simulink model "formation_control_alternative_tanks"  (R2021a)
settings: Solver=VariableStepAuto  StartTime=0.0  StopTime=T  RelTol=1e-3
undefined symbols (not defined in the file or in its folder): params
settings Model: Creator=gaeta  LastModifiedBy=giuse
settings SolverCC: AlgebraicLoopSolver=TrustRegion
settings DataIOCC: InitialState=initialCondition  LoadInitialState=on
settings DebuggingCC: SFMachineParentedDataDiag=warning

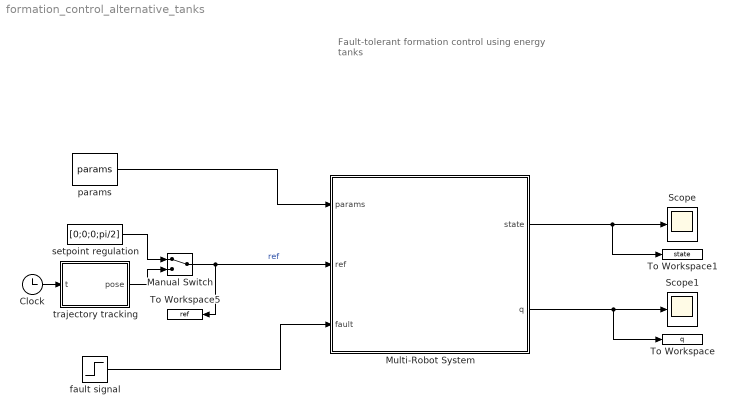
== system formation_control_alternative_tanks ==
  note: Fault-tolerant formation control
      | using energy tanks
  Clock : Clock
  Manual Switch : ManualSwitch
  Multi-Robot System : Subsystem
  Scope : Scope
  Scope1 : Scope
  To Workspace : ToWorkspace  VariableName=q  SaveFormat=Timeseries  SampleTime=-1
  To Workspace1 : ToWorkspace  VariableName=state  SaveFormat=Timeseries  SampleTime=-1
  To Workspace5 : ToWorkspace  VariableName=ref  SaveFormat=Timeseries  SampleTime=-1
  fault signal : Step  Time=25  SampleTime=0
  params : Constant  Value=params  OutDataTypeStr=Bus: params_bus
  setpoint regulation : Constant  Value=[0;0;0;pi/2]
  trajectory tracking : MATLAB Function  TreatAsAtomicUnit=on
  wires:
  trajectory tracking/1(pose) -> Manual Switch/2
  setpoint regulation/1 -> Manual Switch/1
  Clock/1 -> trajectory tracking/1(t)
  Manual Switch/1 -> To Workspace5/1, Multi-Robot System/2(ref)  "ref"
  Multi-Robot System/2(q) -> Scope1/1, To Workspace/1
  Multi-Robot System/1(state) -> Scope/1, To Workspace1/1
  params/1 -> Multi-Robot System/1(params)
  fault signal/1 -> Multi-Robot System/3(fault)

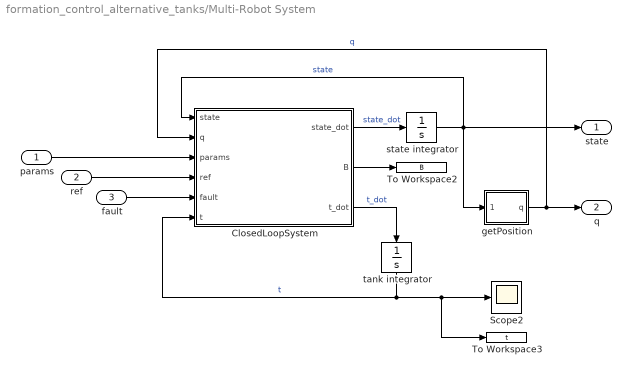
== system formation_control_alternative_tanks/Multi-Robot System ==
  params : Inport
  ref : Inport  Port=2
  fault : Inport  Port=3
  ClosedLoopSystem : MATLAB Function  TreatAsAtomicUnit=on
  Scope2 : Scope
  To Workspace2 : ToWorkspace  VariableName=B  SaveFormat=Timeseries  SampleTime=-1
  To Workspace3 : ToWorkspace  VariableName=t  SaveFormat=Timeseries  SampleTime=-1
  getPosition : Subsystem
  state integrator : Integrator
  tank integrator : Integrator
  state : Outport
  q : Outport  Port=2
  wires:
  ClosedLoopSystem/3(t_dot) -> tank integrator/1  "t_dot"
  getPosition/1(q) -> q/1, ClosedLoopSystem/2(q)  "q"
  ref/1 -> ClosedLoopSystem/4(ref)
  state integrator/1 -> state/1, ClosedLoopSystem/1(state), getPosition/1(state)  "state"
  ClosedLoopSystem/2(B) -> To Workspace2/1
  ClosedLoopSystem/1(state_dot) -> state integrator/1  "state_dot"
  tank integrator/1 -> To Workspace3/1, Scope2/1, ClosedLoopSystem/6(t)  "t"
  fault/1 -> ClosedLoopSystem/5(fault)
  params/1 -> ClosedLoopSystem/3(params)

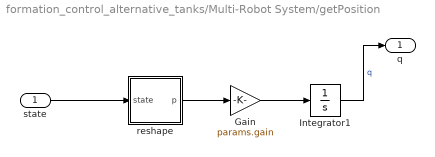
== system formation_control_alternative_tanks/Multi-Robot System/getPosition ==
  state : Inport
  Gain : Gain  Gain=params.gain
  Integrator1 : Integrator
  reshape : MATLAB Function  TreatAsAtomicUnit=on
  q : Outport
  wires:
  state/1 -> reshape/1(state)
  reshape/1(p) -> Gain/1
  Gain/1 -> Integrator1/1
  Integrator1/1 -> q/1  "q"

== matlab function formation_control_alternative_tanks/trajectory tracking ==
  data: pose output size=4; t input size=1
%% generate reference trajectory
function pose = trajectory(t)
t1 = 5;
t_end = 55;

w = 0.25;
phi = -w*t1;
A = 80;
z_vel = 1;

if(t<t1)
    y = [0;0;0];
    theta = pi/2;
elseif(t>t_end)
    y = [A*sin(w*t_end+phi); -A*cos(w*t_end+phi); z_vel*t_end] - [A*sin(w*t1+phi); -A*cos(w*t1+phi); z_vel*t1];
    theta = atan2(A*sin(w*t_end+phi), A*cos(w*t_end+phi));
else
    y = [A*sin(w*t+phi); -A*cos(w*t+phi); z_vel*t] - [A*sin(w*t1+phi); -A*cos(w*t1+phi); z_vel*t1];
    theta = atan2(A*sin(w*t+phi), A*cos(w*t+phi));
end

pose = [y; theta];
end

== matlab function formation_control_alternative_tanks/Multi-Robot System/ClosedLoopSystem ==
  data: state input size=3*(params.N+params.E); q input size=3*params.N; state_dot output size=3*(params.N+params.E); params input; ref input size=4; fault input; t input size=params.N; B output; t_dot output size=params.N
function [state_dot,B,t_dot] = closedLoopSystem(state, q, params, ref, fault, t)
n = 3;	% task space
N = 5;  % number of robots
faulted_robot = params.faulted_robot;
alpha = zeros(N,1);

%% initialize some matrices
p = state(1:n*N);           % robots momenta
m = params.m;               % robots masses
M = zeros(n*N, n*N);      	% inertia matrix
d = params.d;               % frict. coeff
D = zeros(n*N, n*N);        % system dissipation matrix
for i = 1:N
    M(n*i-n+1:n*i, n*i-n+1:n*i) = eye(n).*m(i);
    D(n*i-n+1:n*i, n*i-n+1:n*i) = eye(n).*d(i);
end

%% Check whether a fault is occurred
if(sum(fault)~=0 && ~params.fault_occurred)
    params.fault_occurred = 1;  % flag on
    params.B = faultHandler(params.B, params.Bfull, faulted_robot);
end

%% Still initialize matrices
E = params.E;               % number of edges
B = params.B;
Bcl = kron(params.B,eye(n));% closed-loop incidence matrix
dc = params.dc;             % robots dissipations
Dc = zeros(n*E, n*E);       % controller dissipation matrix
kc = params.kc;             % constant springs
Kc = zeros(n*E, n*E);       % constant spring matrix
R = zeros(n*E, n*E);        % n*E matrix containing E rotation matrices

for j = 1:E
    Dc(n*j-n+1:n*j, n*j-n+1:n*j) = eye(n).*dc(j);
    Kc(n*j-n+1:n*j, n*j-n+1:n*j) = eye(n).*kc(j);
    R(n*j-n+1:n*j, n*j-n+1:n*j) = rotz(ref(4)-pi/2);
end

z = state(n*N+1:n*(N+E));	% edges lengths
z_des = R*params.z_des;     % desired edges lengths

% NOTE: constant matrices M, D, Dc, Kc should be moved in the Init file

%% Trajectory Tracking / Setpoint Regulation
tracking = true;    % #CHANGE THIS: ENABLE/DISABLE TRAJECTORY TRACKING
u = zeros(n*N,1);
if(tracking) 
    % control for leader trajectory tracking
    Kp = 20;
    u(1:n) = Kp*(ref(1:n)-q(1:n));
    
    % control for faulted robot
    K_pd = 0.4;
    P_action = K_pd*(1-q(n*faulted_robot));
	D_action = K_pd*p(n*faulted_robot)/m(faulted_robot);
    u(n*faulted_robot) = params.fault_occurred*(P_action-D_action);
end

%% Multi-robot System Dynamics
Fe = -Bcl * Kc*(z-z_des);           % external forces (control action)
Fa = -(Bcl*Dc*Bcl.')*(M^(-1)*p);	% interaction (coupling) forces
p_dot = Fa + Fe - D*(M^(-1)*p) + u;

% dissipated energy stored in tanks
dissipated_storage = zeros(N,1);
for i = 1:N
    if t(i) >= params.tank_max
        alpha(i) = 0;
    else
        alpha(i) = 1;
    end
    p_i = p(n*i-n+1:i*n);
    M_i = M(n*i-n+1:i*n, n*i-n+1:i*n);
    D_i = D(n*i-n+1:i*n, n*i-n+1:i*n);
    dissipated_storage(i) = alpha(i)*( 1/(t(i)) * ( p_i.' * inv(M_i.') * D_i * inv(M_i) * p_i ) );   
end

% interaction forcess
F = zeros(n,E);
for e = 1:E
    if(isConnected(e,B))
        F(:,e) = kc(e)*( z(n*e-n+1:e*n) - z_des(n*e-n+1:e*n) ); % store force exchanged in edge e-th
    else
        F(:,e) = zeros(n,1);
    end
end

%% Energy transfer protocol
gamma = params.gamma;
t_dot = zeros(N,1);
for i = 1:N
    energy_exchange_tank = 0;
    for e = 1:E
        energy_exchange_tank = energy_exchange_tank + B(i,e)*gamma(e)*t(i)*(F(:,e).'*F(:,e));
    end
    t_dot(i) = dissipated_storage(i) + alpha(i)*energy_exchange_tank;
end

z_dot_a = Bcl.'*(M^(-1)*p);
z_dot_b = zeros(E*n,1);
for e = 1:E
    energy_exchange_spring = zeros(n,1);
    for i = 1:N
        energy_exchange_spring = energy_exchange_spring - B(i,e)*gamma(i)*t(i)^2*F(:,e);
    end
    z_dot_b(e*n-n+1:e*n) = energy_exchange_spring;
end

z_dot = z_dot_a + z_dot_b;

state_dot = [p_dot; z_dot];
end


%% Energy function ----------------------------------------------
function v = V(error)
if (error<=0)
    v = error^2;
elseif(error>=0 && error<5*pi)
    v = 50*cos(0.2*error-pi)+50;
else
    v = 100;
end
end

%% Derivative of the energy function
function vdot = Vdot(error)
if (error<=0)
    vdot = 2*error;
elseif(error>0 && error<5*pi)
    vdot = 10*sin(0.2*error);
else
    vdot = 0;
end
end

%% Split & Join operations
function B = faultHandler(B, Bfull, faulted_robot)
% split procedure
if(faulted_robot==1)
    disp("leader cannot be faulted by hypothesis");
else
    faulted_edges = getEdges(faulted_robot, B);
    for e = 1:size(B,2)
        if(ismember(e,faulted_edges))
           B(:,e) = zeros(size(B,1),1); 
        end
    end
end

% join procedure
if(faulted_robot==size(B,1))
    i = faulted_robot-1;
    j = 1;
else
    i = faulted_robot-1;
    j = faulted_robot+1;
end
joined_edge = getEdge(i,j,Bfull);
B(:,joined_edge) = Bfull(:,joined_edge);
end

% given a robot, return connected edges
function edges = getEdges(robot, B)
edges = find(B(robot,:)~=0);
end

% given 2 robots, return the edge connecting them, 0 otherwise
function edge = getEdge(i, j, B)
edge = 0;
for e = 1:size(B,2)
    if( (B(i,e)==1 && B(j,e)==-1) || (B(i,e)==-1 && B(j,e)==1) )
        edge = e;
        break
    end
end
end

% check whether an edge is connected
function ret = isConnected(e,B)
if(sum(abs(B(:,e)))~=0)
    ret = 1;
else
    ret = 0;
end
end

%

== matlab function formation_control_alternative_tanks/Multi-Robot System/getPosition/reshape ==
  data: p output size=3*params.N; state input size=3*(params.N+params.E)
function p = reshape(state)
    %n = 3;
    %N = roots([n/2, n/2, -size(state,1)]).'*(roots([n/2, n/2, -size(state,1)])>0);
    N = 5;
    p = state(1:3*5);
end




%
